simulink model "ibob_phased_array_2k"  (Simulink 7.0)
settings: Solver=ode45  StartTime=0.0  StopTime=70  RelTol=1e-3
undefined symbols (not defined in the file or in its folder): iBOB
libraries: xbsIndex_r4 x666, xps_library x63, beamform x4, casper_library x3
(part 1 of 6)
settings Model: Creator=Administrator  LastModifiedBy=Administrator
settings DebuggingCC: SaveWithParameterizedLinksMsg=none  SignalResolutionControl=TryResolveAllWithWarning  MultiTaskDSMMsg=warning  MultiTaskCondExecSysMsg=none  StrictBusMsg=None
settings RTWCC: IncludeERTFirstTime=on
settings GRTTargetCC: TargetFcnLib=ansi_tfl_tmw.mat

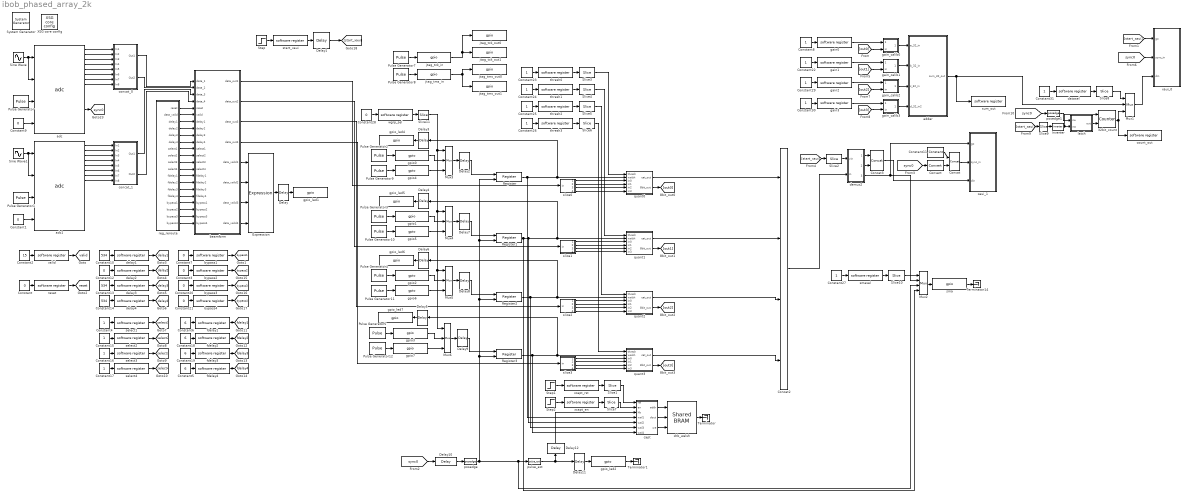
== system ibob_phased_array_2k ==
  " System Generator" : xbsIndex_r4/ System Generator  Tag=genX  SystemSampleTime=-1  xilinxfamily=virtex2p  part=xc2vp50  speed=-7  package=ff1152  synthesis_tool=XST  clock_wrapper=Clock Enables  directory=./ibob_phased_array_2k/sysgen  testbench=off  simulink_period=1  sysclk_period=3.9063  dcm_input_clock_period=100  incr_netlist=off  trim_vbits=Everywhere in SubSystem  dbl_ovrd=According to Block Masks  core_generation=According to Block Masks  run_coregen=off  deprecated_control=off  eval_field=0  block_type=sysgen
      settings: block_version=10.1.3
  32bit_count : xbsIndex_r4/Counter  cnt_type=Free Running  cnt_to=Inf  operation=Up  start_count=0  cnt_by_val=1  arith_type=Unsigned  n_bits=32  bin_pt=0  load_pin=off  rst=on  en=on  explicit_period=on  period=1  dbl_ovrd=off  use_behavioral_HDL=off  use_rpm=on  implementation=Fabric  block_type=counter
      settings: xl_area=[0, 0, 0, 0, 0, 0, 0]
  Concat : xbsIndex_r4/Concat  num_inputs=2  dbl_ovrd=off  block_type=concat
      settings: block_version=10.1.3
  Concat2 : xbsIndex_r4/Concat  num_inputs=4  dbl_ovrd=off  block_type=concat
      settings: block_version=10.1.3
  Concat3 : xbsIndex_r4/Concat  num_inputs=2  dbl_ovrd=off  block_type=concat
      settings: block_version=10.1.3
  Constant{,1,3,7,9,12,20..21,28} (9 alike) : Constant  Value=0  OutDataType=sfix(16)  OutScaling=2^0
  Constant10 : Constant  Value=534  OutDataType=sfix(16)  OutScaling=2^0
  Constant11 : xbsIndex_r4/Constant  arith_type=Unsigned  const=0  n_bits=7  bin_pt=0  explicit_period=on  period=1  equ=P=C  opselect=C  inp2=PCIN>>17  opr=+  inp1=P  carry=CIN  dbl_ovrd=off  block_type=constant
  Constant13 : Constant  Value=534  OutDataType=sfix(16)  OutScaling=2^0
  Constant14 : Constant  Value=534  OutDataType=sfix(16)  OutScaling=2^0
  Constant{4,8,15..17,22..27,29..31} (14 alike) : Constant  OutDataType=sfix(16)  OutScaling=2^0
  Constant{5..6,18..19} (4 alike) : Constant  Value=6  OutDataType=sfix(16)  OutScaling=2^0
  Constant2 : Constant  Value=15  OutDataType=sfix(16)  OutScaling=2^0
  Convert : xbsIndex_r4/Convert  arith_type=Unsigned  n_bits=1  bin_pt=0  quantization=Truncate  overflow=Wrap  latency=0  dbl_ovrd=off  pipeline=off  block_type=convert
      settings: xl_area=[0, 0, 0, 0, 0, 0, 0]  block_version=10.1.3
  Delay : xbsIndex_r4/Delay  en=off  latency=15  dbl_ovrd=off  reg_retiming=off  block_type=delay
      settings: xl_area=[0, 0, 0, 0, 0, 0, 0]
  Delay{1..2,7..9} (5 alike) : xbsIndex_r4/Delay  en=off  latency=10  dbl_ovrd=off  reg_retiming=on  block_type=delay
      settings: xl_area=[0, 0, 0, 0, 0, 0, 0]
  Delay10 : xbsIndex_r4/Delay  en=off  latency=5  dbl_ovrd=off  reg_retiming=on  block_type=delay
      settings: xl_area=[0, 0, 0, 0, 0, 0, 0]
  Delay11 : xbsIndex_r4/Delay  en=off  latency=2  dbl_ovrd=off  reg_retiming=on  block_type=delay
      settings: xl_area=[0, 0, 0, 0, 0, 0, 0]
  Delay12 : xbsIndex_r4/Delay  Orientation=up  en=off  latency=2  dbl_ovrd=off  reg_retiming=on  block_type=delay
      settings: xl_area=[0, 0, 0, 0, 0, 0, 0]
  Delay{3..6} (4 alike) : xbsIndex_r4/Delay  Orientation=left  en=off  latency=16  dbl_ovrd=off  reg_retiming=off  block_type=delay
      settings: xl_area=[0, 0, 0, 0, 0, 0, 0]
  Expression : xbsIndex_r4/Expression  expression=a & b & c & d  align_bp=on  en=off  latency=1  precision=Full  arith_type=Unsigned  n_bits=8  bin_pt=2  dbl_ovrd=off  block_type=expr
      settings: xl_area=[0, 0, 0, 0, 0, 0, 0]  block_version=10.1.3
  Inverter : xbsIndex_r4/Inverter  en=off  latency=0  dbl_ovrd=off  block_type=inv
      settings: xl_area=[0, 0, 0, 0, 0, 0, 0]
  Mux1 : xbsIndex_r4/Mux  inputs=2  en=off  latency=2  precision=Full  arith_type="Signed  (2's comp)"  n_bits=8  bin_pt=2  quantization=Truncate  overflow=Wrap  dbl_ovrd=off  block_type=mux
      settings: xl_area=[0, 0, 0, 0, 0, 0, 0]
  Mux2 : xbsIndex_r4/Mux  inputs=3  en=off  latency=2  precision=Full  arith_type="Signed  (2's comp)"  n_bits=8  bin_pt=2  quantization=Truncate  overflow=Wrap  dbl_ovrd=off  block_type=mux
      settings: xl_area=[0, 0, 0, 0, 0, 0, 0]
  Mux{3..6} (4 alike) : xbsIndex_r4/Mux  inputs=2  en=off  latency=0  precision=Full  arith_type="Signed  (2's comp)"  n_bits=8  bin_pt=2  quantization=Truncate  overflow=Wrap  dbl_ovrd=off  block_type=mux
      settings: xl_area=[0, 0, 0, 0, 0, 0, 0]
  Pulse Generator : DiscretePulseGenerator  Period=100  PulseWidth=20
  Pulse Generator1 : DiscretePulseGenerator  Period=100  PulseWidth=20
  Pulse Generator{3,5,10,12} (4 alike) : DiscretePulseGenerator  Period=200  PulseWidth=100  PhaseDelay=200
  Pulse Generator{2,4,7..9,11} (6 alike) : DiscretePulseGenerator  Period=200  PulseWidth=100
  Register{,1..3} (4 alike) : xbsIndex_r4/Register  init=0  rst=off  en=on  dbl_ovrd=off  block_type=register
      settings: xl_area=[0, 0, 0, 0, 0, 0, 0]
  Sine Wave : Sin  SineType=Sample based  Amplitude=0.9  Frequency=6.4340e+9  Samples=60  SampleTime=1/4
  Sine Wave1 : Sin  SineType=Sample based  Amplitude=0.9  Frequency=6.4340e+9  Samples=60  SampleTime=1/4
  Slice{1..2,7,9} (4 alike) : xbsIndex_r4/Slice  nbits=1  boolean_output=on  mode=Lower Bit Location + Width  bit1=0  base1=MSB of Input  bit0=0  base0=LSB of Input  dbl_ovrd=off  block_type=slice
      settings: infoedit="Extracts a given range of bits from each input sample and presents it at the output.  The output type is ordinarily unsigned with binary point at zero, but can be Boolean when the slice is one bit wide.<P><P>Hardware notes: In hardware this block costs nothing."  block_version=10.1.3
  Slice10 : xbsIndex_r4/Slice  nbits=2  boolean_output=off  mode=Lower Bit Location + Width  bit1=0  base1=MSB of Input  bit0=0  base0=LSB of Input  dbl_ovrd=off  block_type=slice
      settings: infoedit="Extracts a given range of bits from each input sample and presents it at the output.  The output type is ordinarily unsigned with binary point at zero, but can be Boolean when the slice is one bit wide.<P><P>Hardware notes: In hardware this block costs nothing."  block_version=10.1.3
  Slice11 : xbsIndex_r4/Slice  nbits=1  boolean_output=off  mode=Lower Bit Location + Width  bit1=0  base1=MSB of Input  bit0=0  base0=LSB of Input  dbl_ovrd=off  block_type=slice
      settings: infoedit="Extracts a given range of bits from each input sample and presents it at the output.  The output type is ordinarily unsigned with binary point at zero, but can be Boolean when the slice is one bit wide.<P><P>Hardware notes: In hardware this block costs nothing."  block_version=10.1.3
  Slice{3..6} (4 alike) : xbsIndex_r4/Slice  nbits=7  boolean_output=off  mode=Lower Bit Location + Width  bit1=0  base1=MSB of Input  bit0=0  base0=LSB of Input  dbl_ovrd=off  block_type=slice
      settings: infoedit="Extracts a given range of bits from each input sample and presents it at the output.  The output type is ordinarily unsigned with binary point at zero, but can be Boolean when the slice is one bit wide.<P><P>Hardware notes: In hardware this block costs nothing."  block_version=10.1.3
  Slice8 : xbsIndex_r4/Slice  nbits=1  boolean_output=off  mode=Lower Bit Location + Width  bit1=0  base1=MSB of Input  bit0=0  base0=LSB of Input  dbl_ovrd=off  block_type=slice
      settings: infoedit="Extracts a given range of bits from each input sample and presents it at the output.  The output type is ordinarily unsigned with binary point at zero, but can be Boolean when the slice is one bit wide.<P><P>Hardware notes: In hardware this block costs nothing."  block_version=10.1.3
  Step : Step  Time=100  SampleTime=0
  Step1 : Step  Time=100  SampleTime=0
  Step2 : Step  Time=100  SampleTime=0
  Terminator : Terminator
  Terminator1 : Terminator
  Terminator14 : Terminator
  XSG core config : xps_library/XSG core config  Tag=xps:xsg  SystemSampleTime=-1  hw_sys=iBOB  ibob_linux=off  clk_src=adc0_clk  iBOB_clk_src=adc0_clk  BEE2_ctrl_clk_src=sys_clk  BEE2_usr_clk_src=sys_clk  ROACH_clk_src=sys_clk  CORR_clk_src=sys_clk  gpio_clk_io_group=iBOB:sma  gpio_clk_bit_index=0  clk_rate=256  sample_period=1  synthesis_tool=XST  mpc_type=powerpc405
  adc : xps_library/adc  Tag=xps:adc  SystemSampleTime=-1  adc_brd=adc0  adc_clk_rate=1024  adc_interleave=off  sample_period=1
  adc1 : xps_library/adc  Tag=xps:adc  SystemSampleTime=-1  adc_brd=adc1  adc_clk_rate=1024  adc_interleave=off  sample_period=1
  adder : Subsystem
  beamform : Subsystem
  bypass1 : xps_library/software register  Tag=xps:sw_reg  SystemSampleTime=-1  io_dir=From Processor  arith_type=Unsigned  bitwidth=32  bin_pt=0  sample_period=1  gw_name=ibob_phased_array_2k_bypass1_user_data_out
      link override ibob_phased_array_2k_bypass1_user_data_out: arith_type=Unsigned  n_bits=32  bin_pt=0  period=1
  bypass2 : xps_library/software register  Tag=xps:sw_reg  SystemSampleTime=-1  io_dir=From Processor  arith_type=Unsigned  bitwidth=32  bin_pt=0  sample_period=1  gw_name=ibob_phased_array_2k_bypass2_user_data_out
      link override ibob_phased_array_2k_bypass2_user_data_out: arith_type=Unsigned  n_bits=32  bin_pt=0  period=1
  bypass3 : xps_library/software register  Tag=xps:sw_reg  SystemSampleTime=-1  io_dir=From Processor  arith_type=Unsigned  bitwidth=32  bin_pt=0  sample_period=1  gw_name=ibob_phased_array_2k_bypass3_user_data_out
      link override ibob_phased_array_2k_bypass3_user_data_out: arith_type=Unsigned  n_bits=32  bin_pt=0  period=1
  bypass4 : xps_library/software register  Tag=xps:sw_reg  SystemSampleTime=-1  io_dir=From Processor  arith_type=Unsigned  bitwidth=32  bin_pt=0  sample_period=1  gw_name=ibob_phased_array_2k_bypass4_user_data_out
      link override ibob_phased_array_2k_bypass4_user_data_out: arith_type=Unsigned  n_bits=32  bin_pt=0  period=1
  capt : Subsystem
  concat_0 : Subsystem
  concat_1 : Subsystem
  count_out : xps_library/software register  Tag=xps:sw_reg  SystemSampleTime=-1  io_dir=To Processor  arith_type=Unsigned  bitwidth=32  bin_pt=0  sample_period=1  gw_name=ibob_phased_array_2k_count_out_user_data_in
      link override convert: arith_type=Unsigned  n_bits=32  bin_pt=0
  datasel : xps_library/software register  Tag=xps:sw_reg  SystemSampleTime=-1  io_dir=From Processor  arith_type=Unsigned  bitwidth=32  bin_pt=0  sample_period=1  gw_name=ibob_phased_array_2k_datasel_user_data_out
      link override ibob_phased_array_2k_datasel_user_data_out: arith_type=Unsigned  n_bits=32  bin_pt=0  period=1
  delay1 : xps_library/software register  Tag=xps:sw_reg  SystemSampleTime=-1  io_dir=From Processor  arith_type=Unsigned  bitwidth=32  bin_pt=0  sample_period=1  gw_name=ibob_phased_array_2k_delay1_user_data_out
      link override ibob_phased_array_2k_delay1_user_data_out: arith_type=Unsigned  n_bits=32  bin_pt=0  period=1
  delay2 : xps_library/software register  Tag=xps:sw_reg  SystemSampleTime=-1  io_dir=From Processor  arith_type=Unsigned  bitwidth=32  bin_pt=0  sample_period=1  gw_name=ibob_phased_array_2k_delay2_user_data_out
      link override ibob_phased_array_2k_delay2_user_data_out: arith_type=Unsigned  n_bits=32  bin_pt=0  period=1
  delay3 : xps_library/software register  Tag=xps:sw_reg  SystemSampleTime=-1  io_dir=From Processor  arith_type=Unsigned  bitwidth=32  bin_pt=0  sample_period=1  gw_name=ibob_phased_array_2k_delay3_user_data_out
      link override ibob_phased_array_2k_delay3_user_data_out: arith_type=Unsigned  n_bits=32  bin_pt=0  period=1
  delay4 : xps_library/software register  Tag=xps:sw_reg  SystemSampleTime=-1  io_dir=From Processor  arith_type=Unsigned  bitwidth=32  bin_pt=0  sample_period=1  gw_name=ibob_phased_array_2k_delay4_user_data_out
      link override ibob_phased_array_2k_delay4_user_data_out: arith_type=Unsigned  n_bits=32  bin_pt=0  period=1
  demux2 : Subsystem
  fdelay1 : xps_library/software register  Tag=xps:sw_reg  SystemSampleTime=-1  io_dir=From Processor  arith_type=Unsigned  bitwidth=32  bin_pt=0  sample_period=1  gw_name=ibob_phased_array_2k_fdelay1_user_data_out
      link override ibob_phased_array_2k_fdelay1_user_data_out: arith_type=Unsigned  n_bits=32  bin_pt=0  period=1
  fdelay2 : xps_library/software register  Tag=xps:sw_reg  SystemSampleTime=-1  io_dir=From Processor  arith_type=Unsigned  bitwidth=32  bin_pt=0  sample_period=1  gw_name=ibob_phased_array_2k_fdelay2_user_data_out
      link override ibob_phased_array_2k_fdelay2_user_data_out: arith_type=Unsigned  n_bits=32  bin_pt=0  period=1
  fdelay3 : xps_library/software register  Tag=xps:sw_reg  SystemSampleTime=-1  io_dir=From Processor  arith_type=Unsigned  bitwidth=32  bin_pt=0  sample_period=1  gw_name=ibob_phased_array_2k_fdelay3_user_data_out
      link override ibob_phased_array_2k_fdelay3_user_data_out: arith_type=Unsigned  n_bits=32  bin_pt=0  period=1
  fdelay4 : xps_library/software register  Tag=xps:sw_reg  SystemSampleTime=-1  io_dir=From Processor  arith_type=Unsigned  bitwidth=32  bin_pt=0  sample_period=1  gw_name=ibob_phased_array_2k_fdelay4_user_data_out
      link override ibob_phased_array_2k_fdelay4_user_data_out: arith_type=Unsigned  n_bits=32  bin_pt=0  period=1
  gain0 : xps_library/software register  Tag=xps:sw_reg  SystemSampleTime=-1  io_dir=From Processor  arith_type="Signed  (2's comp)"  bitwidth=32  bin_pt=7  sample_period=1  gw_name=ibob_phased_array_2k_gain0_user_data_out
      link override ibob_phased_array_2k_gain0_user_data_out: arith_type="Signed  (2's comp)"  n_bits=32  bin_pt=7  period=1
  gain1 : xps_library/software register  Tag=xps:sw_reg  SystemSampleTime=-1  io_dir=From Processor  arith_type="Signed  (2's comp)"  bitwidth=32  bin_pt=7  sample_period=1  gw_name=ibob_phased_array_2k_gain1_user_data_out
      link override ibob_phased_array_2k_gain1_user_data_out: arith_type="Signed  (2's comp)"  n_bits=32  bin_pt=7  period=1
  gain2 : xps_library/software register  Tag=xps:sw_reg  SystemSampleTime=-1  io_dir=From Processor  arith_type="Signed  (2's comp)"  bitwidth=32  bin_pt=7  sample_period=1  gw_name=ibob_phased_array_2k_gain2_user_data_out
      link override ibob_phased_array_2k_gain2_user_data_out: arith_type="Signed  (2's comp)"  n_bits=32  bin_pt=7  period=1
  gain3 : xps_library/software register  Tag=xps:sw_reg  SystemSampleTime=-1  io_dir=From Processor  arith_type="Signed  (2's comp)"  bitwidth=32  bin_pt=7  sample_period=1  gw_name=ibob_phased_array_2k_gain3_user_data_out
      link override ibob_phased_array_2k_gain3_user_data_out: arith_type="Signed  (2's comp)"  n_bits=32  bin_pt=7  period=1
  gain_calib0 : Subsystem
  gain_calib1 : Subsystem
  gain_calib2 : Subsystem
  gain_calib3 : Subsystem
  gpio0 : xps_library/gpio  Tag=xps:gpio  SystemSampleTime=-1  io_group=iBOB:gpio0  io_dir=in  arith_type=Boolean  bitwidth=1  bin_pt=0  bit_index=0  sample_period=1  use_single_ended=off  use_ddr=off  reg_iob=on  reg_clk_phase=0  termination=None
      link override ibob_phased_array_2k_gpio0_gateway: arith_type=Boolean  n_bits=1  bin_pt=0  period=sample_period
  gpio1 : xps_library/gpio  Tag=xps:gpio  SystemSampleTime=-1  io_group=iBOB:gpio0  io_dir=in  arith_type=Boolean  bitwidth=1  bin_pt=0  bit_index=1  sample_period=1  use_single_ended=off  use_ddr=off  reg_iob=on  reg_clk_phase=0  termination=None
      link override ibob_phased_array_2k_gpio1_gateway: arith_type=Boolean  n_bits=1  bin_pt=0  period=sample_period
  gpio2 : xps_library/gpio  Tag=xps:gpio  SystemSampleTime=-1  io_group=iBOB:gpio0  io_dir=in  arith_type=Boolean  bitwidth=1  bin_pt=0  bit_index=2  sample_period=1  use_single_ended=off  use_ddr=off  reg_iob=on  reg_clk_phase=0  termination=None
      link override ibob_phased_array_2k_gpio2_gateway: arith_type=Boolean  n_bits=1  bin_pt=0  period=sample_period
  gpio3 : xps_library/gpio  Tag=xps:gpio  SystemSampleTime=-1  io_group=iBOB:gpio0  io_dir=in  arith_type=Boolean  bitwidth=1  bin_pt=0  bit_index=3  sample_period=1  use_single_ended=off  use_ddr=off  reg_iob=on  reg_clk_phase=0  termination=None
      link override ibob_phased_array_2k_gpio3_gateway: arith_type=Boolean  n_bits=1  bin_pt=0  period=sample_period
  gpio4 : xps_library/gpio  Tag=xps:gpio  SystemSampleTime=-1  io_group=iBOB:gpio0  io_dir=in  arith_type=Boolean  bitwidth=1  bin_pt=0  bit_index=4  sample_period=1  use_single_ended=off  use_ddr=off  reg_iob=on  reg_clk_phase=0  termination=None
      link override ibob_phased_array_2k_gpio4_gateway: arith_type=Boolean  n_bits=1  bin_pt=0  period=sample_period
  gpio5 : xps_library/gpio  Tag=xps:gpio  SystemSampleTime=-1  io_group=iBOB:gpio0  io_dir=in  arith_type=Boolean  bitwidth=1  bin_pt=0  bit_index=5  sample_period=1  use_single_ended=off  use_ddr=off  reg_iob=on  reg_clk_phase=0  termination=None
      link override ibob_phased_array_2k_gpio5_gateway: arith_type=Boolean  n_bits=1  bin_pt=0  period=sample_period
  gpio6 : xps_library/gpio  Tag=xps:gpio  SystemSampleTime=-1  io_group=iBOB:gpio0  io_dir=in  arith_type=Boolean  bitwidth=1  bin_pt=0  bit_index=6  sample_period=1  use_single_ended=off  use_ddr=off  reg_iob=on  reg_clk_phase=0  termination=None
      link override ibob_phased_array_2k_gpio6_gateway: arith_type=Boolean  n_bits=1  bin_pt=0  period=sample_period
  gpio7 : xps_library/gpio  Tag=xps:gpio  SystemSampleTime=-1  io_group=iBOB:gpio0  io_dir=in  arith_type=Boolean  bitwidth=1  bin_pt=0  bit_index=7  sample_period=1  use_single_ended=off  use_ddr=off  reg_iob=on  reg_clk_phase=0  termination=None
      link override ibob_phased_array_2k_gpio7_gateway: arith_type=Boolean  n_bits=1  bin_pt=0  period=sample_period
  gpio_led1 : xps_library/gpio  Tag=xps:gpio  SystemSampleTime=-1  io_group=iBOB:led  io_dir=out  arith_type=Boolean  bitwidth=1  bin_pt=0  bit_index=1  sample_period=1  use_single_ended=off  use_ddr=off  reg_iob=on  reg_clk_phase=0  termination=None
      link override convert: arith_type=Boolean  n_bits=1  bin_pt=0
  gpio_led2 : xps_library/gpio  Tag=xps:gpio  SystemSampleTime=-1  io_group=iBOB:led  io_dir=out  arith_type=Boolean  bitwidth=1  bin_pt=0  bit_index=2  sample_period=1  use_single_ended=off  use_ddr=off  reg_iob=on  reg_clk_phase=0  termination=None
      link override convert: arith_type=Boolean  n_bits=1  bin_pt=0
  gpio_led4 : xps_library/gpio  Tag=xps:gpio  Orientation=left  SystemSampleTime=-1  io_group=iBOB:led  io_dir=out  arith_type=Boolean  bitwidth=1  bin_pt=0  bit_index=4  sample_period=1  use_single_ended=off  use_ddr=off  reg_iob=on  reg_clk_phase=0  termination=None
      link override convert: arith_type=Boolean  n_bits=1  bin_pt=0
  gpio_led5 : xps_library/gpio  Tag=xps:gpio  Orientation=left  SystemSampleTime=-1  io_group=iBOB:led  io_dir=out  arith_type=Boolean  bitwidth=1  bin_pt=0  bit_index=5  sample_period=1  use_single_ended=off  use_ddr=off  reg_iob=on  reg_clk_phase=0  termination=None
      link override convert: arith_type=Boolean  n_bits=1  bin_pt=0
  gpio_led6 : xps_library/gpio  Tag=xps:gpio  Orientation=left  SystemSampleTime=-1  io_group=iBOB:led  io_dir=out  arith_type=Boolean  bitwidth=1  bin_pt=0  bit_index=6  sample_period=1  use_single_ended=off  use_ddr=off  reg_iob=on  reg_clk_phase=0  termination=None
      link override convert: arith_type=Boolean  n_bits=1  bin_pt=0
  gpio_led7 : xps_library/gpio  Tag=xps:gpio  Orientation=left  SystemSampleTime=-1  io_group=iBOB:led  io_dir=out  arith_type=Boolean  bitwidth=1  bin_pt=0  bit_index=7  sample_period=1  use_single_ended=off  use_ddr=off  reg_iob=on  reg_clk_phase=0  termination=None
      link override convert: arith_type=Boolean  n_bits=1  bin_pt=0
  jtag_tck_in : xps_library/gpio  Tag=xps:gpio  SystemSampleTime=-1  io_group=iBOB:gpio1  io_dir=in  arith_type=Boolean  bitwidth=1  bin_pt=0  bit_index=0  sample_period=1  use_single_ended=off  use_ddr=off  reg_iob=on  reg_clk_phase=0  termination=None
      link override ibob_phased_array_2k_jtag_tck_in_gateway: arith_type=Boolean  n_bits=1  bin_pt=0  period=sample_period
  jtag_tck_out0 : xps_library/gpio  Tag=xps:gpio  SystemSampleTime=-1  io_group=iBOB:gpio1  io_dir=out  arith_type=Boolean  bitwidth=1  bin_pt=0  bit_index=2  sample_period=1  use_single_ended=off  use_ddr=off  reg_iob=on  reg_clk_phase=0  termination=None
      link override convert: arith_type=Boolean  n_bits=1  bin_pt=0
  jtag_tck_out1 : xps_library/gpio  Tag=xps:gpio  SystemSampleTime=-1  io_group=iBOB:gpio1  io_dir=out  arith_type=Boolean  bitwidth=1  bin_pt=0  bit_index=3  sample_period=1  use_single_ended=off  use_ddr=off  reg_iob=on  reg_clk_phase=0  termination=None
      link override convert: arith_type=Boolean  n_bits=1  bin_pt=0
  jtag_tms_in : xps_library/gpio  Tag=xps:gpio  SystemSampleTime=-1  io_group=iBOB:gpio1  io_dir=in  arith_type=Boolean  bitwidth=1  bin_pt=0  bit_index=1  sample_period=1  use_single_ended=off  use_ddr=off  reg_iob=on  reg_clk_phase=0  termination=None
      link override ibob_phased_array_2k_jtag_tms_in_gateway: arith_type=Boolean  n_bits=1  bin_pt=0  period=sample_period
  jtag_tms_out0 : xps_library/gpio  Tag=xps:gpio  SystemSampleTime=-1  io_group=iBOB:gpio1  io_dir=out  arith_type=Boolean  bitwidth=1  bin_pt=0  bit_index=4  sample_period=1  use_single_ended=off  use_ddr=off  reg_iob=on  reg_clk_phase=0  termination=None
      link override convert: arith_type=Boolean  n_bits=1  bin_pt=0
  jtag_tms_out1 : xps_library/gpio  Tag=xps:gpio  SystemSampleTime=-1  io_group=iBOB:gpio1  io_dir=out  arith_type=Boolean  bitwidth=1  bin_pt=0  bit_index=5  sample_period=1  use_single_ended=off  use_ddr=off  reg_iob=on  reg_clk_phase=0  termination=None
      link override convert: arith_type=Boolean  n_bits=1  bin_pt=0
  latch : Subsystem
  posedge : casper_library/Misc/posedge  Tag=Rising Edge Detector  SystemSampleTime=-1
  posedge1 : casper_library/Misc/posedge  Tag=Rising Edge Detector  SystemSampleTime=-1
  pulse_ext : casper_library/Misc/pulse_ext  SystemSampleTime=-1  pulse_len=20000*32
  quant0 : Subsystem
  quant1 : Subsystem
  quant2 : Subsystem
  quant3 : Subsystem
  reg_reroute : Subsystem
  reset : xps_library/software register  Tag=xps:sw_reg  SystemSampleTime=-1  io_dir=From Processor  arith_type=Unsigned  bitwidth=32  bin_pt=0  sample_period=1  gw_name=ibob_phased_array_2k_reset_user_data_out
      link override ibob_phased_array_2k_reset_user_data_out: arith_type=Unsigned  n_bits=32  bin_pt=0  period=1
  select1 : xps_library/software register  Tag=xps:sw_reg  SystemSampleTime=-1  io_dir=From Processor  arith_type=Unsigned  bitwidth=32  bin_pt=0  sample_period=1  gw_name=ibob_phased_array_2k_select1_user_data_out
      link override ibob_phased_array_2k_select1_user_data_out: arith_type=Unsigned  n_bits=32  bin_pt=0  period=1
  select2 : xps_library/software register  Tag=xps:sw_reg  SystemSampleTime=-1  io_dir=From Processor  arith_type=Unsigned  bitwidth=32  bin_pt=0  sample_period=1  gw_name=ibob_phased_array_2k_select2_user_data_out
      link override ibob_phased_array_2k_select2_user_data_out: arith_type=Unsigned  n_bits=32  bin_pt=0  period=1
  select3 : xps_library/software register  Tag=xps:sw_reg  SystemSampleTime=-1  io_dir=From Processor  arith_type=Unsigned  bitwidth=32  bin_pt=0  sample_period=1  gw_name=ibob_phased_array_2k_select3_user_data_out
      link override ibob_phased_array_2k_select3_user_data_out: arith_type=Unsigned  n_bits=32  bin_pt=0  period=1
  select4 : xps_library/software register  Tag=xps:sw_reg  SystemSampleTime=-1  io_dir=From Processor  arith_type=Unsigned  bitwidth=32  bin_pt=0  sample_period=1  gw_name=ibob_phased_array_2k_select4_user_data_out
      link override ibob_phased_array_2k_select4_user_data_out: arith_type=Unsigned  n_bits=32  bin_pt=0  period=1
  slice0 : Subsystem
  slice1 : Subsystem
  slice2 : Subsystem
  slice3 : Subsystem
  sma : xps_library/gpio  Tag=xps:gpio  SystemSampleTime=-1  io_group=iBOB:sma  io_dir=out  arith_type=Boolean  bitwidth=1  bin_pt=0  bit_index=1  sample_period=1  use_single_ended=off  use_ddr=off  reg_iob=on  reg_clk_phase=0  termination=None
      link override convert: arith_type=Boolean  n_bits=1  bin_pt=0
  smasel : xps_library/software register  Tag=xps:sw_reg  SystemSampleTime=-1  io_dir=From Processor  arith_type=Unsigned  bitwidth=32  bin_pt=0  sample_period=1  gw_name=ibob_phased_array_2k_smasel_user_data_out
      link override ibob_phased_array_2k_smasel_user_data_out: arith_type=Unsigned  n_bits=32  bin_pt=0  period=1
  start_xaui : xps_library/software register  Tag=xps:sw_reg  SystemSampleTime=-1  io_dir=From Processor  arith_type=Unsigned  bitwidth=32  bin_pt=0  sample_period=1  gw_name=ibob_phased_array_2k_start_xaui_user_data_out
      link override ibob_phased_array_2k_start_xaui_user_data_out: arith_type=Unsigned  n_bits=32  bin_pt=0  period=1
  sum_out : xps_library/software register  Tag=xps:sw_reg  SystemSampleTime=-1  io_dir=To Processor  arith_type=Unsigned  bitwidth=32  bin_pt=0  sample_period=1  gw_name=ibob_phased_array_2k_sum_out_user_data_in
      link override convert: arith_type=Unsigned  n_bits=32  bin_pt=0
  thresh0 : xps_library/software register  Tag=xps:sw_reg  SystemSampleTime=-1  io_dir=From Processor  arith_type=Unsigned  bitwidth=32  bin_pt=0  sample_period=1  gw_name=ibob_phased_array_2k_thresh0_user_data_out
      link override ibob_phased_array_2k_thresh0_user_data_out: arith_type=Unsigned  n_bits=32  bin_pt=0  period=1
  thresh1 : xps_library/software register  Tag=xps:sw_reg  SystemSampleTime=-1  io_dir=From Processor  arith_type=Unsigned  bitwidth=32  bin_pt=0  sample_period=1  gw_name=ibob_phased_array_2k_thresh1_user_data_out
      link override ibob_phased_array_2k_thresh1_user_data_out: arith_type=Unsigned  n_bits=32  bin_pt=0  period=1
  thresh2 : xps_library/software register  Tag=xps:sw_reg  SystemSampleTime=-1  io_dir=From Processor  arith_type=Unsigned  bitwidth=32  bin_pt=0  sample_period=1  gw_name=ibob_phased_array_2k_thresh2_user_data_out
      link override ibob_phased_array_2k_thresh2_user_data_out: arith_type=Unsigned  n_bits=32  bin_pt=0  period=1
  thresh3 : xps_library/software register  Tag=xps:sw_reg  SystemSampleTime=-1  io_dir=From Processor  arith_type=Unsigned  bitwidth=32  bin_pt=0  sample_period=1  gw_name=ibob_phased_array_2k_thresh3_user_data_out
      link override ibob_phased_array_2k_thresh3_user_data_out: arith_type=Unsigned  n_bits=32  bin_pt=0  period=1
  valid : xps_library/software register  Tag=xps:sw_reg  SystemSampleTime=-1  io_dir=From Processor  arith_type=Unsigned  bitwidth=32  bin_pt=0  sample_period=1  gw_name=ibob_phased_array_2k_valid_user_data_out
      link override ibob_phased_array_2k_valid_user_data_out: arith_type=Unsigned  n_bits=32  bin_pt=0  period=1
  wgrp_sel : xps_library/software register  Tag=xps:sw_reg  SystemSampleTime=-1  io_dir=From Processor  arith_type=Unsigned  bitwidth=32  bin_pt=0  sample_period=1  gw_name=ibob_phased_array_2k_wgrp_sel_user_data_out
      link override ibob_phased_array_2k_wgrp_sel_user_data_out: arith_type=Unsigned  n_bits=32  bin_pt=0  period=1
  xaui_0 : Subsystem
  xaui_1 : Subsystem
  xcapt_en : xps_library/software register  Tag=xps:sw_reg  SystemSampleTime=-1  io_dir=From Processor  arith_type=Unsigned  bitwidth=32  bin_pt=0  sample_period=1  gw_name=ibob_phased_array_2k_xcapt_en_user_data_out
      link override ibob_phased_array_2k_xcapt_en_user_data_out: arith_type=Unsigned  n_bits=32  bin_pt=0  period=1
  xcapt_rst : xps_library/software register  Tag=xps:sw_reg  SystemSampleTime=-1  io_dir=From Processor  arith_type=Unsigned  bitwidth=32  bin_pt=0  sample_period=1  gw_name=ibob_phased_array_2k_xcapt_rst_user_data_out
      link override ibob_phased_array_2k_xcapt_rst_user_data_out: arith_type=Unsigned  n_bits=32  bin_pt=0  period=1
  xhb_walsh : xps_library/Shared BRAM  Tag=xps:bram  SystemSampleTime=-1  arith_type=Unsigned  addr_width=13  data_width=32  data_bin_pt=0  init_vals=[1:2^13]  sample_rate=1
      link override convert_din: arith_type=Unsigned
      link override ibob_phased_array_2k_xhb_walsh_data_out: arith_type=Unsigned
      link override mem/sim_data_in: arith_type=Unsigned
  tag scope: bypass1=global, bypass2=global, bypass3=global, bypass4=global, delay1=global, delay2=global, delay3=global, delay4=global, fdelay1=global, fdelay2=global, fdelay3=global, fdelay4=global, reset=global, select1=global, select2=global, select3=global, select4=global, sync0=global, valid=global
  wires:
  Constant9/1 -> adc/4
  Constant1/1 -> adc1/4
  beamform/5(data_valid1) -> Expression/1
  beamform/6(data_valid2) -> Expression/2
  beamform/7(data_valid3) -> Expression/3
  beamform/8(data_valid4) -> Expression/4
  Delay/1 -> gpio_led1/1
  Constant/1 -> reset/1
  Constant7/1 -> bypass1/1
  Constant12/1 -> delay2/1
  Constant13/1 -> delay3/1
  Constant14/1 -> delay4/1
  Constant4/1 -> select1/1
  Constant15/1 -> select2/1
  Constant16/1 -> select3/1
  Constant17/1 -> select4/1
  Constant6/1 -> fdelay1/1
  Constant18/1 -> fdelay2/1
  Constant19/1 -> fdelay3/1
  Constant5/1 -> fdelay4/1
  bypass1/1 -> [bypass1]
  reset/1 -> [reset]
  delay2/1 -> [delay2]
  delay3/1 -> [delay3]
  delay4/1 -> [delay4]
  select1/1 -> [select1]
  select2/1 -> [select2]
  select3/1 -> [select3]
  select4/1 -> [select4]
  fdelay1/1 -> [fdelay1]
  fdelay2/1 -> [fdelay2]
  fdelay3/1 -> [fdelay3]
  fdelay4/1 -> [fdelay4]
  Expression/1 -> Delay/1
  Sine Wave1/1 -> adc1/1, adc1/2
  Sine Wave/1 -> adc/1, adc/2
  Constant10/1 -> delay1/1
  delay1/1 -> [delay1]
  Constant2/1 -> valid/1
  valid/1 -> [valid]
  Constant3/1 -> bypass2/1
  bypass2/1 -> [bypass2]
  Constant20/1 -> bypass3/1
  bypass3/1 -> [bypass3]
  Constant21/1 -> bypass4/1
  bypass4/1 -> [bypass4]
  reg_reroute/1(reset) -> beamform/5(reset)
  reg_reroute/2(data_valid) -> beamform/6(valid)
  reg_reroute/3(delay1) -> beamform/7(delay1)
  reg_reroute/4(delay2) -> beamform/8(delay2)
  reg_reroute/5(delay3) -> beamform/9(delay3)
  reg_reroute/6(delay4) -> beamform/10(delay4)
  reg_reroute/7(select1) -> beamform/11(select1)
  reg_reroute/8(select2) -> beamform/12(select2)
  reg_reroute/9(select3) -> beamform/13(select3)
  reg_reroute/10(select4) -> beamform/14(select4)
  reg_reroute/11(fdelay1) -> beamform/15(fdelay1)
  reg_reroute/12(fdelay2) -> beamform/16(fdelay2)
  reg_reroute/13(fdelay3) -> beamform/17(fdelay3)
  reg_reroute/14(fdelay4) -> beamform/18(fdelay4)
  reg_reroute/15(bypass1) -> beamform/19(bypass1)
  reg_reroute/16(bypass2) -> beamform/20(bypass2)
  reg_reroute/17(bypass3) -> beamform/21(bypass3)
  reg_reroute/18(bypass4) -> beamform/22(bypass4)
  concat_0/1(Out1) -> beamform/1(data_1)
  concat_0/2(Out2) -> beamform/2(data_2)
  concat_1/1(Out1) -> beamform/3(data_3)
  concat_1/2(Out2) -> beamform/4(data_4)
  Pulse Generator/1 -> adc/3
  Pulse Generator1/1 -> adc1/3
  Step/1 -> start_xaui/1
  start_xaui/1 -> Delay1/1
  Delay1/1 -> [start_xaui]
  demux2/3(valid) -> xaui_1/1(go), Mux2/2
  adc/13 -> [sync0]
  demux2/1(out0) -> Concat3/1
  demux2/2(out1) -> Concat3/2
  Slice2/1 -> demux2/1(vin)
  [start_xaui] -> Slice2/1
  thresh0/1 -> Slice3/1
  Constant23/1 -> thresh0/1
  thresh1/1 -> Slice4/1
  Constant24/1 -> thresh1/1
  thresh2/1 -> Slice5/1
  Constant25/1 -> thresh2/1
  thresh3/1 -> Slice6/1
  Constant26/1 -> thresh3/1
  quant0/1(cat_out) -> Concat2/1
  quant1/1(cat_out) -> Concat2/2
  quant2/1(cat_out) -> Concat2/3
  quant3/1(cat_out) -> Concat2/4
  Concat2/1 -> demux2/2(in)
  sma/1 -> Terminator14/1
  Pulse Generator3/1 -> gpio1/1
  Delay4/1 -> gpio_led5/1
  adc/1 -> concat_0/1(In1)
  adc/2 -> concat_0/2(In2)
  adc/3 -> concat_0/3(In3)
  adc/4 -> concat_0/4(In4)
  adc/5 -> concat_0/5(In5)
  adc/6 -> concat_0/6(In6)
  adc/7 -> concat_0/7(In7)
  adc/8 -> concat_0/8(In8)
  adc1/1 -> concat_1/1(In1)
  adc1/2 -> concat_1/2(In2)
  adc1/3 -> concat_1/3(In3)
  adc1/4 -> concat_1/4(In4)
  adc1/5 -> concat_1/5(In5)
  adc1/6 -> concat_1/6(In6)
  adc1/7 -> concat_1/7(In7)
  adc1/8 -> concat_1/8(In8)
  Pulse Generator4/1 -> gpio2/1
  Pulse Generator5/1 -> gpio3/1
  Delay5/1 -> gpio_led7/1
  Delay6/1 -> gpio_led6/1
  Slice3/1 -> quant0/1(thresh)
  Slice4/1 -> quant1/1(thresh)
  Slice5/1 -> quant2/1(thresh)
  Slice6/1 -> quant3/1(thresh)
  beamform/1(data_out1) -> slice0/1(in)
  beamform/2(data_out2) -> slice1/1(in)
  beamform/3(data_out3) -> slice2/1(in)
  beamform/4(data_out4) -> slice3/1(in)
  Pulse Generator2/1 -> gpio0/1
  Delay3/1 -> gpio_led4/1
  slice0/1(out0) -> quant0/3(in0)
  slice0/2(out1) -> quant0/4(in1)
  slice0/3(out2) -> quant0/5(in2)
  slice0/4(out3) -> quant0/6(in3)
  slice1/1(out0) -> quant1/3(in0)
  slice1/2(out1) -> quant1/4(in1)
  slice1/3(out2) -> quant1/5(in2)
  slice1/4(out3) -> quant1/6(in3)
  slice2/1(out0) -> quant2/3(in0)
  slice2/2(out1) -> quant2/4(in1)
  slice2/3(out2) -> quant2/5(in2)
  slice2/4(out3) -> quant2/6(in3)
  slice3/1(out0) -> quant3/3(in0)
  slice3/2(out1) -> quant3/4(in1)
  slice3/3(out2) -> quant3/5(in2)
  slice3/4(out3) -> quant3/6(in3)
  Register/1 -> quant0/2(walsh), Delay3/1, capt/4(wal1)
  Register1/1 -> Mux2/4, Delay4/1, quant1/2(walsh), capt/5(wal2)
  Register2/1 -> Delay6/1, quant2/2(walsh), capt/6(wal3)
  Register3/1 -> Delay5/1, quant3/2(walsh), capt/7(wal4)
  [sync0] -> Delay10/1
  Delay10/1 -> posedge/1
  [sync0] -> Convert/1
  Concat/1 -> xaui_1/2(sync_in)
  Constant11/1 -> Concat/1
  Convert/1 -> Concat/2
  gpio_led2/1 -> Terminator1/1
  Mux2/1 -> sma/1
  smasel/1 -> Slice10/1
  Constant27/1 -> smasel/1
  Slice10/1 -> Mux2/1
  posedge/1 -> Mux2/3, pulse_ext/1, Register3/2, Register2/2, Register1/2, Register/2
  pulse_ext/1 -> Delay11/1, Delay12/1
  Pulse Generator7/1 -> jtag_tck_in/1
  Pulse Generator8/1 -> jtag_tms_in/1
  jtag_tck_in/1 -> jtag_tck_out0/1, jtag_tck_out1/1
  jtag_tms_in/1 -> jtag_tms_out0/1, jtag_tms_out1/1
  quant0/2(8bit_out) -> [out0]
  quant1/2(8bit_out) -> [out1]
  quant2/2(8bit_out) -> [out2]
  quant3/2(8bit_out) -> [out3]
  Pulse Generator9/1 -> gpio4/1
  gpio0/1 -> Mux3/2
  gpio4/1 -> Mux3/3
  Pulse Generator10/1 -> gpio5/1
  gpio1/1 -> Mux4/2
  gpio5/1 -> Mux4/3
  Pulse Generator11/1 -> gpio6/1
  gpio2/1 -> Mux5/2
  gpio6/1 -> Mux5/3
  Mux3/1 -> Delay2/1
  Mux4/1 -> Delay7/1
  Mux5/1 -> Delay8/1
  Pulse Generator12/1 -> gpio7/1
  gpio3/1 -> Mux6/2
  gpio7/1 -> Mux6/3
  Mux6/1 -> Delay9/1
  Constant28/1 -> wgrp_sel/1
  wgrp_sel/1 -> Slice11/1
  Slice11/1 -> Mux3/1, Mux4/1, Mux5/1, Mux6/1
  adder/1(sum_32_out) -> sum_out/1, Mux1/2
  [start_xaui] -> xaui_0/1(go)
  [sync0] -> xaui_0/2(sync_in)
  gain0/1 -> gain_calib0/1(gain)
  Constant8/1 -> gain0/1
  gain1/1 -> gain_calib1/1(gain)
  Constant22/1 -> gain1/1
  gain2/1 -> gain_calib2/1(gain)
  Constant29/1 -> gain2/1
  gain3/1 -> gain_calib3/1(gain)
  Constant30/1 -> gain3/1
  gain_calib0/1(out) -> adder/1(a_32_in)
  gain_calib1/1(out) -> adder/2(b_32_in)
  gain_calib2/1(out) -> adder/3(c_32_in)
  gain_calib3/1(out) -> adder/4(d_32_in2)
  [out0] -> gain_calib0/2(in)
  [out1] -> gain_calib1/2(in)
  [out2] -> gain_calib2/2(in)
  [out3] -> gain_calib3/2(in)
  Delay2/1 -> Register/1
  Delay7/1 -> Register1/1
  Delay8/1 -> Register2/1
  Delay9/1 -> Register3/1
  Delay11/1 -> gpio_led2/1
  xhb_walsh/1 -> Terminator/1
  capt/1(addr) -> xhb_walsh/1
  capt/3(we) -> xhb_walsh/3
  capt/2(dout) -> xhb_walsh/2
  xcapt_rst/1 -> Slice1/1
  Step1/1 -> xcapt_rst/1
  Step2/1 -> xcapt_en/1
  xcapt_en/1 -> Slice7/1
  Slice1/1 -> capt/1(rst)
  Slice7/1 -> capt/2(en)
  datasel/1 -> Slice8/1
  Constant31/1 -> datasel/1
  Slice8/1 -> Mux1/1
  latch/1(out) -> 32bit_count/2
  32bit_count/1 -> count_out/1, Mux1/3
  [start_xaui] -> Slice9/1
  Inverter/1 -> latch/2(rst), 32bit_count/1
  [sync0] -> posedge1/1
  posedge1/1 -> latch/1(sw)
  Slice9/1 -> Inverter/1
  Concat3/1 -> xaui_1/3(din)
  Mux1/1 -> xaui_0/3(din)
  Delay12/1 -> capt/3(hb)

== system ibob_phased_array_2k/adder ==
  a_32_in : Inport  OutDataType=sfix(16)  OutScaling=2^0
  b_32_in : Inport  Port=2  OutDataType=sfix(16)  OutScaling=2^0
  c_32_in : Inport  Port=3  OutDataType=sfix(16)  OutScaling=2^0
  d_32_in2 : Inport  Port=4  OutDataType=sfix(16)  OutScaling=2^0
  Subsystem : Subsystem
  Subsystem1 : Subsystem
  Subsystem2 : Subsystem
  sum_32_out : Outport  OutDataType=sfix(16)  OutScaling=2^0
  wires:
  Subsystem1/1(Out1) -> Subsystem2/2(b_32_in)
  Subsystem/1(Out1) -> Subsystem2/1(a_32_in)
  d_32_in2/1 -> Subsystem1/2(b_32_in)
  c_32_in/1 -> Subsystem1/1(a_32_in)
  b_32_in/1 -> Subsystem/2(b_32_in)
  a_32_in/1 -> Subsystem/1(a_32_in)
  Subsystem2/1(Out1) -> sum_32_out/1

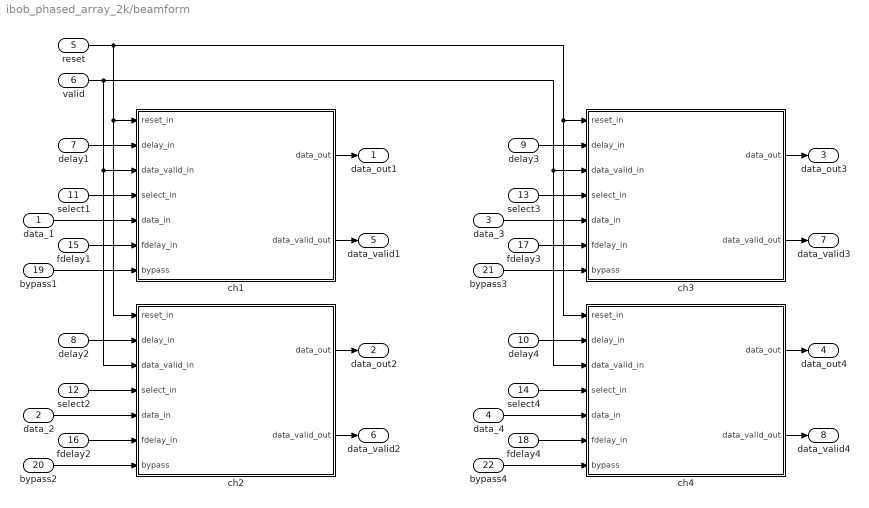
== system ibob_phased_array_2k/beamform ==
  data_1 : Inport  OutDataType=sfix(16)  OutScaling=2^0
  data_2 : Inport  Port=2  OutDataType=sfix(16)  OutScaling=2^0
  data_3 : Inport  Port=3  OutDataType=sfix(16)  OutScaling=2^0
  data_4 : Inport  Port=4  OutDataType=sfix(16)  OutScaling=2^0
  reset : Inport  Port=5  OutDataType=sfix(16)  OutScaling=2^0
  valid : Inport  Port=6  OutDataType=sfix(16)  OutScaling=2^0
  delay1 : Inport  Port=7  OutDataType=sfix(16)  OutScaling=2^0
  delay2 : Inport  Port=8  OutDataType=sfix(16)  OutScaling=2^0
  delay3 : Inport  Port=9  OutDataType=sfix(16)  OutScaling=2^0
  delay4 : Inport  Port=10  OutDataType=sfix(16)  OutScaling=2^0
  select1 : Inport  Port=11  OutDataType=sfix(16)  OutScaling=2^0
  select2 : Inport  Port=12  OutDataType=sfix(16)  OutScaling=2^0
  select3 : Inport  Port=13  OutDataType=sfix(16)  OutScaling=2^0
  select4 : Inport  Port=14  OutDataType=sfix(16)  OutScaling=2^0
  fdelay1 : Inport  Port=15  OutDataType=sfix(16)  OutScaling=2^0
  fdelay2 : Inport  Port=16  OutDataType=sfix(16)  OutScaling=2^0
  fdelay3 : Inport  Port=17  OutDataType=sfix(16)  OutScaling=2^0
  fdelay4 : Inport  Port=18  OutDataType=sfix(16)  OutScaling=2^0
  bypass1 : Inport  Port=19  OutDataType=sfix(16)  OutScaling=2^0
  bypass2 : Inport  Port=20  OutDataType=sfix(16)  OutScaling=2^0
  bypass3 : Inport  Port=21  OutDataType=sfix(16)  OutScaling=2^0
  bypass4 : Inport  Port=22  OutDataType=sfix(16)  OutScaling=2^0
  ch1 : Subsystem
  ch2 : Subsystem
  ch3 : Subsystem
  ch4 : Subsystem
  data_out1 : Outport  OutDataType=sfix(16)  OutScaling=2^0
  data_out2 : Outport  Port=2  OutDataType=sfix(16)  OutScaling=2^0
  data_out3 : Outport  Port=3  OutDataType=sfix(16)  OutScaling=2^0
  data_out4 : Outport  Port=4  OutDataType=sfix(16)  OutScaling=2^0
  data_valid1 : Outport  Port=5  OutDataType=sfix(16)  OutScaling=2^0
  data_valid2 : Outport  Port=6  OutDataType=sfix(16)  OutScaling=2^0
  data_valid3 : Outport  Port=7  OutDataType=sfix(16)  OutScaling=2^0
  data_valid4 : Outport  Port=8  OutDataType=sfix(16)  OutScaling=2^0
  wires:
  ch1/1(data_out) -> data_out1/1
  ch1/2(data_valid_out) -> data_valid1/1
  data_2/1 -> ch2/5(data_in)
  data_3/1 -> ch3/5(data_in)
  data_4/1 -> ch4/5(data_in)
  ch2/1(data_out) -> data_out2/1
  ch3/1(data_out) -> data_out3/1
  ch4/1(data_out) -> data_out4/1
  ch2/2(data_valid_out) -> data_valid2/1
  ch3/2(data_valid_out) -> data_valid3/1
  ch4/2(data_valid_out) -> data_valid4/1
  data_1/1 -> ch1/5(data_in)
  delay1/1 -> ch1/2(delay_in)
  delay2/1 -> ch2/2(delay_in)
  delay3/1 -> ch3/2(delay_in)
  delay4/1 -> ch4/2(delay_in)
  reset/1 -> ch1/1(reset_in), ch2/1(reset_in), ch3/1(reset_in), ch4/1(reset_in)
  valid/1 -> ch3/3(data_valid_in), ch4/3(data_valid_in), ch1/3(data_valid_in), ch2/3(data_valid_in)
  select1/1 -> ch1/4(select_in)
  select4/1 -> ch4/4(select_in)
  fdelay1/1 -> ch1/6(fdelay_in)
  select3/1 -> ch3/4(select_in)
  fdelay3/1 -> ch3/6(fdelay_in)
  select2/1 -> ch2/4(select_in)
  fdelay2/1 -> ch2/6(fdelay_in)
  fdelay4/1 -> ch4/6(fdelay_in)
  bypass2/1 -> ch2/7(bypass)
  bypass1/1 -> ch1/7(bypass)
  bypass3/1 -> ch3/7(bypass)
  bypass4/1 -> ch4/7(bypass)

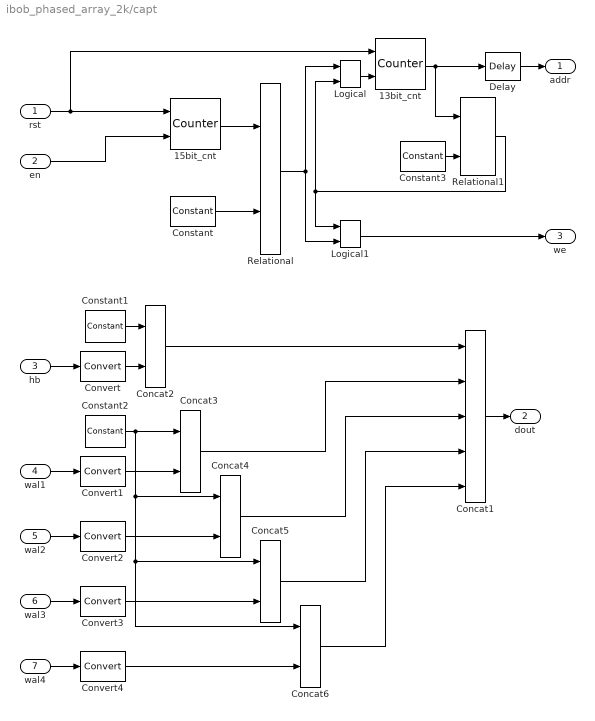
== system ibob_phased_array_2k/capt ==
  rst : Inport  OutDataType=sfix(16)  OutScaling=2^0
  en : Inport  Port=2  OutDataType=sfix(16)  OutScaling=2^0
  hb : Inport  Port=3  OutDataType=sfix(16)  OutScaling=2^0
  wal1 : Inport  Port=4  OutDataType=sfix(16)  OutScaling=2^0
  wal2 : Inport  Port=5  OutDataType=sfix(16)  OutScaling=2^0
  wal3 : Inport  Port=6  OutDataType=sfix(16)  OutScaling=2^0
  wal4 : Inport  Port=7  OutDataType=sfix(16)  OutScaling=2^0
  13bit_cnt : xbsIndex_r4/Counter  cnt_type=Free Running  cnt_to=Inf  operation=Up  start_count=0  cnt_by_val=1  arith_type=Unsigned  n_bits=13  bin_pt=0  load_pin=off  rst=on  en=on  explicit_period=on  period=1  dbl_ovrd=off  use_behavioral_HDL=off  use_rpm=on  implementation=Fabric  block_type=counter
      settings: xl_area=[0, 0, 0, 0, 0, 0, 0]
  15bit_cnt : xbsIndex_r4/Counter  cnt_type=Count Limited  cnt_to=19999  operation=Up  start_count=0  cnt_by_val=1  arith_type=Unsigned  n_bits=15  bin_pt=0  load_pin=off  rst=on  en=on  explicit_period=off  period=1  dbl_ovrd=off  use_behavioral_HDL=off  use_rpm=on  implementation=Fabric  block_type=counter
      settings: xl_area=[0, 0, 0, 0, 0, 0, 0]
  Concat1 : xbsIndex_r4/Concat  num_inputs=5  dbl_ovrd=off  block_type=concat
      settings: block_version=10.1.3
  Concat{2..6} (5 alike) : xbsIndex_r4/Concat  num_inputs=2  dbl_ovrd=off  block_type=concat
      settings: block_version=10.1.3
  Constant : xbsIndex_r4/Constant  arith_type=Unsigned  const=19999  n_bits=15  bin_pt=0  explicit_period=on  period=1  equ=P=C  opselect=C  inp2=PCIN>>17  opr=+  inp1=P  carry=CIN  dbl_ovrd=off  block_type=constant
  Constant1 : xbsIndex_r4/Constant  arith_type=Unsigned  const=0  n_bits=3  bin_pt=0  explicit_period=on  period=1  equ=P=C  opselect=C  inp2=PCIN>>17  opr=+  inp1=P  carry=CIN  dbl_ovrd=off  block_type=constant
  Constant2 : xbsIndex_r4/Constant  arith_type=Unsigned  const=0  n_bits=6  bin_pt=0  explicit_period=on  period=1  equ=P=C  opselect=C  inp2=PCIN>>17  opr=+  inp1=P  carry=CIN  dbl_ovrd=off  block_type=constant
  Constant3 : xbsIndex_r4/Constant  arith_type=Unsigned  const=2^13 -1  n_bits=13  bin_pt=0  explicit_period=on  period=1  equ=P=C  opselect=C  inp2=PCIN>>17  opr=+  inp1=P  carry=CIN  dbl_ovrd=off  block_type=constant
  Convert{,1..4} (5 alike) : xbsIndex_r4/Convert  arith_type=Unsigned  n_bits=1  bin_pt=0  quantization=Truncate  overflow=Wrap  latency=0  dbl_ovrd=off  pipeline=off  block_type=convert
      settings: xl_area=[0, 0, 0, 0, 0, 0, 0]  block_version=10.1.3
  Delay : xbsIndex_r4/Delay  en=off  latency=1  dbl_ovrd=off  reg_retiming=off  block_type=delay
      settings: xl_area=[0, 0, 0, 0, 0, 0, 0]
  Logical : xbsIndex_r4/Logical  logical_function=AND  inputs=2  en=off  latency=0  precision=Full  arith_type=Unsigned  n_bits=8  bin_pt=2  align_bp=on  dbl_ovrd=off  block_type=logical
      settings: xl_area=[0, 0, 0, 0, 0, 0, 0]
  Logical1 : xbsIndex_r4/Logical  logical_function=AND  inputs=2  en=off  latency=0  precision=Full  arith_type=Unsigned  n_bits=8  bin_pt=2  align_bp=on  dbl_ovrd=off  block_type=logical
      settings: xl_area=[0, 0, 0, 0, 0, 0, 0]
  Relational : xbsIndex_r4/Relational  mode=a=b  en=off  latency=1  dbl_ovrd=off  block_type=relational
      settings: xl_area=[0, 0, 0, 0, 0, 0, 0]  block_version=10.1.3
  Relational1 : xbsIndex_r4/Relational  mode=a<b  en=off  latency=1  dbl_ovrd=off  block_type=relational
      settings: xl_area=[0, 0, 0, 0, 0, 0, 0]  block_version=10.1.3
  addr : Outport  OutDataType=sfix(16)  OutScaling=2^0
  dout : Outport  Port=2  OutDataType=sfix(16)  OutScaling=2^0
  we : Outport  Port=3  OutDataType=sfix(16)  OutScaling=2^0
  wires:
  15bit_cnt/1 -> Relational/1
  Constant/1 -> Relational/2
  Relational/1 -> Logical/1, Logical1/2
  13bit_cnt/1 -> Delay/1, Relational1/1
  Delay/1 -> addr/1
  rst/1 -> 13bit_cnt/1, 15bit_cnt/1
  en/1 -> 15bit_cnt/2
  Concat1/1 -> dout/1
  wal1/1 -> Convert1/1
  wal2/1 -> Convert2/1
  wal3/1 -> Convert3/1
  wal4/1 -> Convert4/1
  hb/1 -> Convert/1
  Constant1/1 -> Concat2/1
  Convert/1 -> Concat2/2
  Constant2/1 -> Concat3/1, Concat4/1, Concat5/1, Concat6/1
  Convert1/1 -> Concat3/2
  Convert2/1 -> Concat4/2
  Convert3/1 -> Concat5/2
  Convert4/1 -> Concat6/2
  Concat2/1 -> Concat1/1
  Concat3/1 -> Concat1/2
  Concat4/1 -> Concat1/3
  Concat5/1 -> Concat1/4
  Concat6/1 -> Concat1/5
  Constant3/1 -> Relational1/2
  Logical/1 -> 13bit_cnt/2
  Relational1/1 -> Logical/2, Logical1/1
  Logical1/1 -> we/1

== system ibob_phased_array_2k/concat_0 ==
  In1 : Inport  OutDataType=sfix(16)  OutScaling=2^0
  In2 : Inport  Port=2  OutDataType=sfix(16)  OutScaling=2^0
  In3 : Inport  Port=3  OutDataType=sfix(16)  OutScaling=2^0
  In4 : Inport  Port=4  OutDataType=sfix(16)  OutScaling=2^0
  In5 : Inport  Port=5  OutDataType=sfix(16)  OutScaling=2^0
  In6 : Inport  Port=6  OutDataType=sfix(16)  OutScaling=2^0
  In7 : Inport  Port=7  OutDataType=sfix(16)  OutScaling=2^0
  In8 : Inport  Port=8  OutDataType=sfix(16)  OutScaling=2^0
  Concat : xbsIndex_r4/Concat  num_inputs=4  dbl_ovrd=off  block_type=concat
      settings: block_version=10.1.3
  Concat1 : xbsIndex_r4/Concat  num_inputs=4  dbl_ovrd=off  block_type=concat
      settings: block_version=10.1.3
  Reinterpret{1..8} (8 alike) : xbsIndex_r4/Reinterpret  force_arith_type=on  arith_type=Unsigned  force_bin_pt=on  bin_pt=0  block_type=reinterpret
      settings: infoedit="Changes signal type without altering the binary representation.   You can changed the signal between signed and unsigned, and relocate the binary point.<P><P>Hardware notes: In hardware this block costs nothing.<P><P>Example:  Suppose the input is 6 bits wide, signed, with 2 fractional bits, and the output is forced to unsigned with 0 fractional bits.  Then an input of -2.0 (1110.00 in binary 2's complement) becomes an output of 56 (111000 in binary)."  block_version=10.1.3
  Out1 : Outport  OutDataType=sfix(16)  OutScaling=2^0
  Out2 : Outport  Port=2  OutDataType=sfix(16)  OutScaling=2^0
  wires:
  Reinterpret1/1 -> Concat/2
  Reinterpret2/1 -> Concat/1
  Reinterpret3/1 -> Concat/3
  Reinterpret4/1 -> Concat/4
  Reinterpret5/1 -> Concat1/1
  Reinterpret6/1 -> Concat1/2
  Reinterpret7/1 -> Concat1/3
  Reinterpret8/1 -> Concat1/4
  In1/1 -> Reinterpret2/1
  In2/1 -> Reinterpret1/1
  Concat/1 -> Out1/1
  In3/1 -> Reinterpret3/1
  In4/1 -> Reinterpret4/1
  In5/1 -> Reinterpret5/1
  In6/1 -> Reinterpret6/1
  Concat1/1 -> Out2/1
  In7/1 -> Reinterpret7/1
  In8/1 -> Reinterpret8/1

== system ibob_phased_array_2k/concat_1 ==
  In1 : Inport  OutDataType=sfix(16)  OutScaling=2^0
  In2 : Inport  Port=2  OutDataType=sfix(16)  OutScaling=2^0
  In3 : Inport  Port=3  OutDataType=sfix(16)  OutScaling=2^0
  In4 : Inport  Port=4  OutDataType=sfix(16)  OutScaling=2^0
  In5 : Inport  Port=5  OutDataType=sfix(16)  OutScaling=2^0
  In6 : Inport  Port=6  OutDataType=sfix(16)  OutScaling=2^0
  In7 : Inport  Port=7  OutDataType=sfix(16)  OutScaling=2^0
  In8 : Inport  Port=8  OutDataType=sfix(16)  OutScaling=2^0
  Concat : xbsIndex_r4/Concat  num_inputs=4  dbl_ovrd=off  block_type=concat
      settings: block_version=10.1.3
  Concat1 : xbsIndex_r4/Concat  num_inputs=4  dbl_ovrd=off  block_type=concat
      settings: block_version=10.1.3
  Reinterpret{1..8} (8 alike) : xbsIndex_r4/Reinterpret  force_arith_type=on  arith_type=Unsigned  force_bin_pt=on  bin_pt=0  block_type=reinterpret
      settings: infoedit="Changes signal type without altering the binary representation.   You can changed the signal between signed and unsigned, and relocate the binary point.<P><P>Hardware notes: In hardware this block costs nothing.<P><P>Example:  Suppose the input is 6 bits wide, signed, with 2 fractional bits, and the output is forced to unsigned with 0 fractional bits.  Then an input of -2.0 (1110.00 in binary 2's complement) becomes an output of 56 (111000 in binary)."  block_version=10.1.3
  Out1 : Outport  OutDataType=sfix(16)  OutScaling=2^0
  Out2 : Outport  Port=2  OutDataType=sfix(16)  OutScaling=2^0
  wires:
  In8/1 -> Reinterpret8/1
  In7/1 -> Reinterpret7/1
  Concat1/1 -> Out2/1
  In6/1 -> Reinterpret6/1
  In5/1 -> Reinterpret5/1
  In4/1 -> Reinterpret4/1
  In3/1 -> Reinterpret3/1
  Concat/1 -> Out1/1
  In2/1 -> Reinterpret1/1
  In1/1 -> Reinterpret2/1
  Reinterpret8/1 -> Concat1/4
  Reinterpret7/1 -> Concat1/3
  Reinterpret6/1 -> Concat1/2
  Reinterpret5/1 -> Concat1/1
  Reinterpret4/1 -> Concat/4
  Reinterpret3/1 -> Concat/3
  Reinterpret2/1 -> Concat/1
  Reinterpret1/1 -> Concat/2
